simulink model "Super_twisting"  (R2016b)
settings: Solver=FixedStepAuto  StartTime=0.0  StopTime=100  FixedStep=Ts  RelTol=1e-3
undefined symbols (not defined in the file): DiscIntNeverNeededParam, down, gamma, Kx, lambda, Ts, up, W
libraries: simulink x3
settings Model: Creator=Ashraf  LastModifiedBy=Ashraf

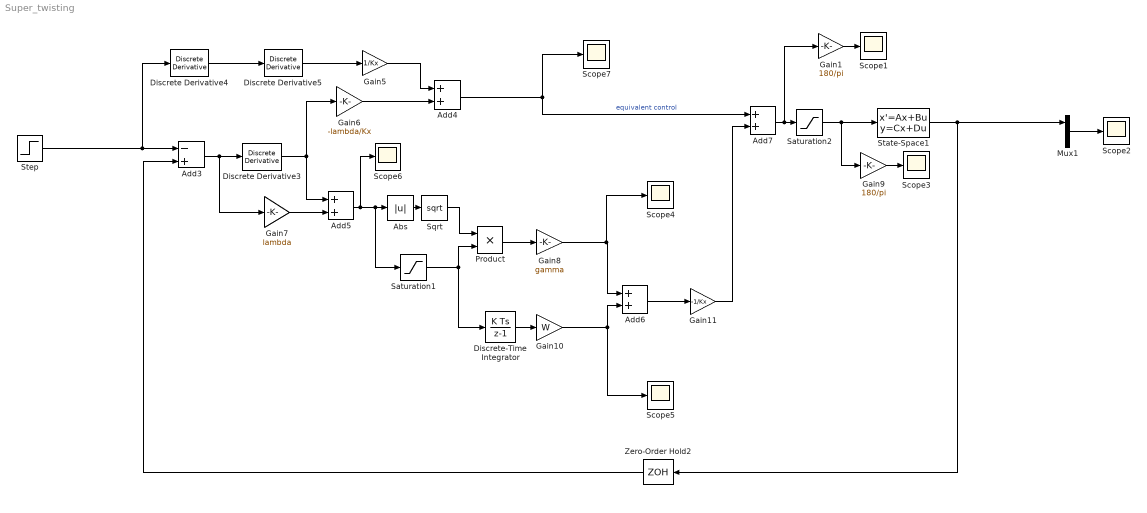
== system Super_twisting ==
  Abs : Abs
  Add3 : Sum  Inputs=-+
  Add{4..7} (4 alike) : Sum
  Discrete Derivative3 : simulink/Discrete/Discrete Derivative  gainval=1.0  ICPrevScaledInput=0.0  OutMin=[]  OutMax=[]  OutDataType=fixdt(1, 16)  OutScaling=2^-10  DoSatur=off
  Discrete Derivative4 : simulink/Discrete/Discrete Derivative  gainval=1.0  ICPrevScaledInput=0.0  OutMin=[]  OutMax=[]  OutDataType=fixdt(1, 16)  OutScaling=2^-10  DoSatur=off
  Discrete Derivative5 : simulink/Discrete/Discrete Derivative  gainval=1.0  ICPrevScaledInput=0.0  OutMin=[]  OutMax=[]  OutDataType=fixdt(1, 16)  OutScaling=2^-10  DoSatur=off
  Discrete-Time Integrator : DiscreteIntegrator  InitialConditionSetting=State (most efficient)  SampleTime=Ts  ICPrevOutput=DiscIntNeverNeededParam  ICPrevScaledInput=DiscIntNeverNeededParam
  Gain1 : Gain  Gain=180/pi
  Gain10 : Gain  Gain=W
  Gain11 : Gain  Gain=-1/Kx
  Gain5 : Gain  Gain=1/Kx
  Gain6 : Gain  Gain=-lambda/Kx
  Gain7 : Gain  Gain=lambda
  Gain8 : Gain  Gain=gamma
  Gain9 : Gain  Gain=180/pi
  Mux1 : Mux  Inputs=2
  Product : Product
  Saturation1 : Saturate  UpperLimit=0.03  LowerLimit=-0.03
  Saturation2 : Saturate  UpperLimit=up  LowerLimit=down
  Scope{1..7} (7 alike) : Scope
  Sqrt : Sqrt  SaturateOnIntegerOverflow=on
  State-Space1 : StateSpace  A=[0 1;0 0]  B=[0;Kx]  C=[1 0]  D=0  X0=[0 0]
  Step : Step  Time=0  After=0.2  SampleTime=Ts
  Zero-Order Hold2 : ZeroOrderHold  SampleTime=Ts
  wires:
  Discrete Derivative5/1 -> Gain5/1
  Add3/1 -> Gain7/1, Discrete Derivative3/1
  Gain5/1 -> Add4/1
  Gain6/1 -> Add4/2
  Discrete Derivative3/1 -> Add5/1, Gain6/1
  State-Space1/1 -> Mux1/1, Zero-Order Hold2/1
  Gain9/1 -> Scope3/1
  Step/1 -> Add3/1, Discrete Derivative4/1
  Mux1/1 -> Scope2/1
  Discrete Derivative4/1 -> Discrete Derivative5/1
  Add7/1 -> Gain1/1, Saturation2/1
  Zero-Order Hold2/1 -> Add3/2
  Gain7/1 -> Add5/2
  Add5/1 -> Scope6/1, Saturation1/1, Abs/1
  Abs/1 -> Sqrt/1
  Sqrt/1 -> Product/1
  Saturation1/1 -> Discrete-Time Integrator/1, Product/2
  Product/1 -> Gain8/1
  Discrete-Time Integrator/1 -> Gain10/1
  Gain8/1 -> Scope4/1, Add6/1
  Gain10/1 -> Scope5/1, Add6/2
  Add6/1 -> Gain11/1
  Add4/1 -> Scope7/1, Add7/1  "equivalent control"
  Gain11/1 -> Add7/2
  Saturation2/1 -> State-Space1/1, Gain9/1
  Gain1/1 -> Scope1/1
